simulink model "UKF"  (R2012b)
settings: Solver=ode4  StartTime=0.0  StopTime=SimulStop  FixedStep=T  RelTol=1e-3
values from neighbouring files (symbols this model uses):
  SimulStop = length(obv_traj1)*T    [parameter_IMM_UKF.m]
  T1 = 0.5    [parameter_IMM_UKF.m]
libraries: commnoisgen2 x1
settings Model: Creator=DonghanLee  LastModifiedBy=DonghanLee

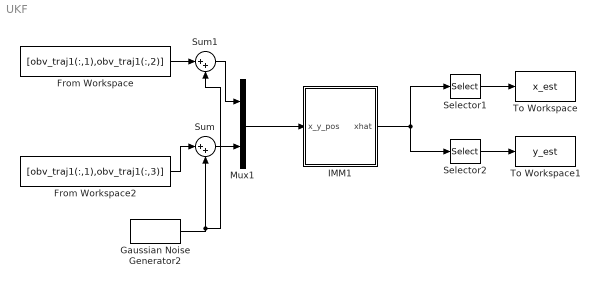
== system UKF ==
  From Workspace : FromWorkspace  VariableName=[obv_traj1(:,1),obv_traj1(:,2)]  SampleTime=0
  From Workspace2 : FromWorkspace  VariableName=[obv_traj1(:,1),obv_traj1(:,3)]  SampleTime=0
  Gaussian Noise Generator2 : commnoisgen2/Gaussian Noise Generator  m=0  d=noise  s=0  Ts=0.05  frameBased=off  sampPerFrame=1  orient=off  outDataType=double
  IMM1 : Subsystem
  Mux1 : Mux  Inputs=2
  Selector1 : Selector  InputPortWidth=5  IndexOptions=Index vector (dialog)  Indices=[1 2]  OutputSizes=1
  Selector2 : Selector  InputPortWidth=5  IndexOptions=Index vector (dialog)  Indices=[3 4]  OutputSizes=1
  Sum : Sum  Inputs=|++
  Sum1 : Sum  Inputs=|++
  To Workspace : ToWorkspace  VariableName=x_est  SampleTime=-1
  To Workspace1 : ToWorkspace  VariableName=y_est  SampleTime=-1
  wires:
  Gaussian Noise Generator2/1 -> Sum1/2, Sum/2
  From Workspace2/1 -> Sum/1
  Sum/1 -> Mux1/2
  From Workspace/1 -> Sum1/1
  Sum1/1 -> Mux1/1
  Mux1/1 -> IMM1/1(x_y_pos)
  IMM1/1(xhat) -> Selector2/1, Selector1/1
  Selector1/1 -> To Workspace/1
  Selector2/1 -> To Workspace1/1

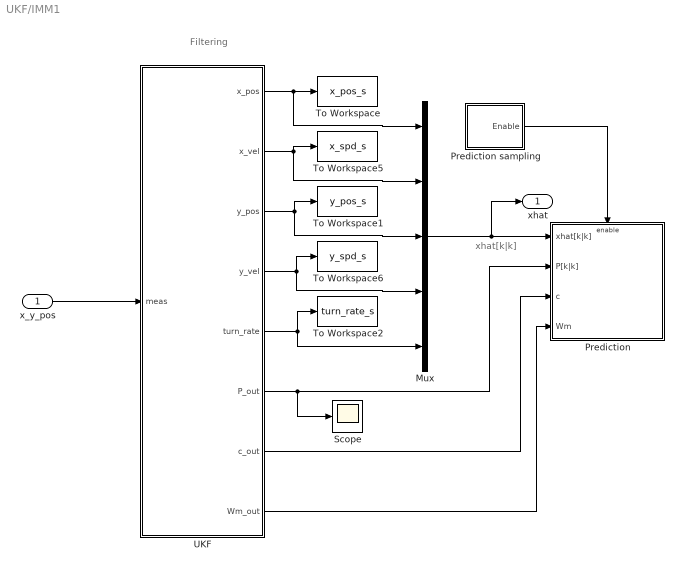
== system UKF/IMM1 ==
  note: xhat[k|k]
  note: Filtering
  x_y_pos : Inport
  Mux : Mux  Inputs=5
  Prediction : Subsystem
  Prediction sampling : Subsystem
  Scope : Scope
      settings: SaveName=ScopeData3
  To Workspace : ToWorkspace  VariableName=x_pos_s  SampleTime=-1
  To Workspace1 : ToWorkspace  VariableName=y_pos_s  SampleTime=-1
  To Workspace2 : ToWorkspace  VariableName=turn_rate_s  SampleTime=-1
  To Workspace5 : ToWorkspace  VariableName=x_spd_s  SampleTime=-1
  To Workspace6 : ToWorkspace  VariableName=y_spd_s  SampleTime=-1
  UKF : MATLAB Function  TreatAsAtomicUnit=on
  xhat : Outport
  wires:
  x_y_pos/1 -> UKF/1(meas)
  UKF/1(x_pos) -> Mux/1, To Workspace/1
  UKF/2(x_vel) -> To Workspace5/1, Mux/2
  UKF/3(y_pos) -> To Workspace1/1, Mux/3
  UKF/4(y_vel) -> To Workspace6/1, Mux/4
  UKF/5(turn_rate) -> To Workspace2/1, Mux/5
  Mux/1 -> xhat/1, Prediction/1(xhat[k|k])
  Prediction sampling/1(Enable) -> Prediction/Enable
  UKF/6(P_out) -> Prediction/2(P[k|k]), Scope/1
  UKF/7(c_out) -> Prediction/3(c)
  UKF/8(Wm_out) -> Prediction/4(Wm)

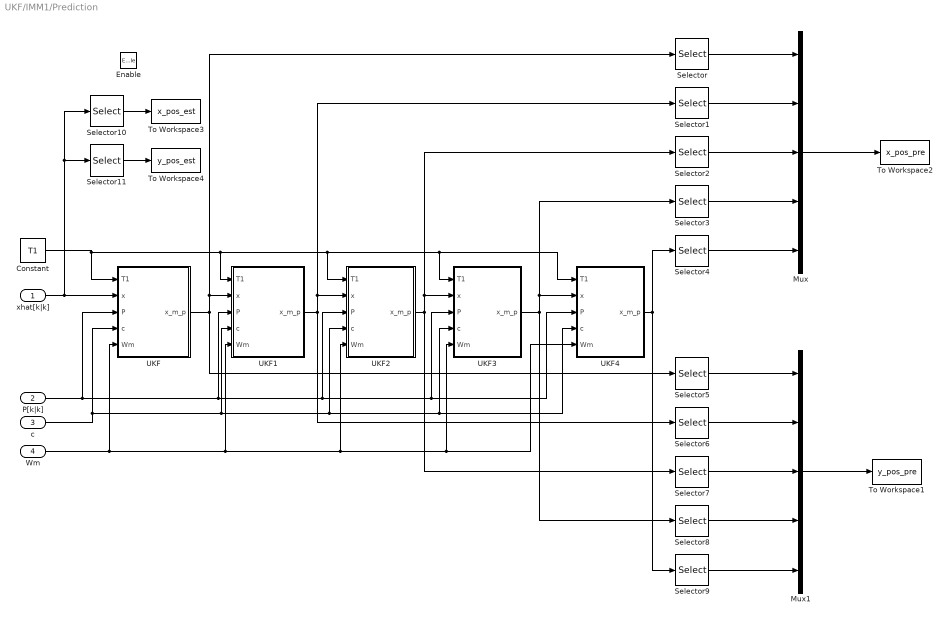
== system UKF/IMM1/Prediction ==
  xhat[k|k] : Inport
  P[k|k] : Inport  Port=2
  c : Inport  Port=3
  Wm : Inport  Port=4
  Enable : EnablePort
  Constant : Constant  Value=T1
  Mux : Mux  Inputs=5
  Mux1 : Mux  Inputs=5
  Selector{,1..4,10} (6 alike) : Selector  InputPortWidth=5  IndexOptions=Index vector (dialog)  Indices=[1]  OutputSizes=1
  Selector{5..9,11} (6 alike) : Selector  InputPortWidth=5  IndexOptions=Index vector (dialog)  Indices=[3]  OutputSizes=1
  To Workspace1 : ToWorkspace  VariableName=y_pos_pre  SampleTime=-1
  To Workspace2 : ToWorkspace  VariableName=x_pos_pre  SampleTime=-1
  To Workspace3 : ToWorkspace  VariableName=x_pos_est  SampleTime=-1
  To Workspace4 : ToWorkspace  VariableName=y_pos_est  SampleTime=-1
  UKF : MATLAB Function  TreatAsAtomicUnit=on
  UKF1 : MATLAB Function  TreatAsAtomicUnit=on
  UKF2 : MATLAB Function  TreatAsAtomicUnit=on
  UKF3 : MATLAB Function  TreatAsAtomicUnit=on
  UKF4 : MATLAB Function  TreatAsAtomicUnit=on
  wires:
  Mux/1 -> To Workspace2/1
  Mux1/1 -> To Workspace1/1
  Selector/1 -> Mux/1
  xhat[k|k]/1 -> UKF/2(x), Selector10/1, Selector11/1
  UKF/1(x_m_p) -> Selector5/1, UKF1/2(x), Selector/1
  UKF1/1(x_m_p) -> Selector6/1, UKF2/2(x), Selector1/1
  UKF2/1(x_m_p) -> Selector7/1, UKF3/2(x), Selector2/1
  UKF3/1(x_m_p) -> Selector8/1, UKF4/2(x), Selector3/1
  UKF4/1(x_m_p) -> Selector9/1, Selector4/1
  Selector2/1 -> Mux/3
  Selector4/1 -> Mux/5
  Selector1/1 -> Mux/2
  Selector3/1 -> Mux/4
  Selector6/1 -> Mux1/2
  Selector8/1 -> Mux1/4
  Selector5/1 -> Mux1/1
  Selector7/1 -> Mux1/3
  Selector9/1 -> Mux1/5
  Selector10/1 -> To Workspace3/1
  Selector11/1 -> To Workspace4/1
  P[k|k]/1 -> UKF1/3(P), UKF2/3(P), UKF4/3(P), UKF3/3(P), UKF/3(P)
  c/1 -> UKF1/4(c), UKF2/4(c), UKF4/4(c), UKF3/4(c), UKF/4(c)
  Wm/1 -> UKF1/5(Wm), UKF2/5(Wm), UKF4/5(Wm), UKF3/5(Wm), UKF/5(Wm)
  Constant/1 -> UKF1/1(T1), UKF2/1(T1), UKF4/1(T1), UKF3/1(T1), UKF/1(T1)

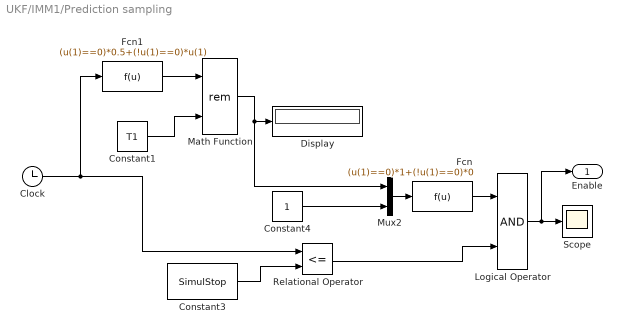
== system UKF/IMM1/Prediction sampling ==
  Clock : Clock
  Constant1 : Constant  Value=T1
  Constant3 : Constant  Value=SimulStop
  Constant4 : Constant
  Display : Display
  Fcn : Fcn  Expr=(u(1)==0)*1+(!u(1)==0)*0
  Fcn1 : Fcn  Expr=(u(1)==0)*0.5+(!u(1)==0)*u(1)
  Logical Operator : Logic  AllPortsSameDT=off  OutDataTypeStr=boolean
  Math Function : Math  Operator=rem  SaturateOnIntegerOverflow=on
  Mux2 : Mux  Inputs=2
  Relational Operator : RelationalOperator  Operator=<=  OutDataTypeStr=boolean
  Scope : Scope
      settings: SaveName=ScopeData2
  Enable : Outport
  wires:
  Clock/1 -> Fcn1/1, Relational Operator/1
  Constant1/1 -> Math Function/2
  Math Function/1 -> Mux2/1, Display/1
  Logical Operator/1 -> Enable/1, Scope/1
  Fcn/1 -> Logical Operator/1
  Relational Operator/1 -> Logical Operator/2
  Constant3/1 -> Relational Operator/2
  Constant4/1 -> Mux2/2
  Mux2/1 -> Fcn/1
  Fcn1/1 -> Math Function/1

== matlab function UKF/IMM1/UKF ==
  data: meas input; x_pos output; x_vel output; y_pos output; y_vel output; turn_rate output; P_out output; c_out output; Wm_out output
function [x_pos,x_vel,y_pos,y_vel,turn_rate,P_out,c_out,Wm_out] = UKF(meas)
% Define parametersInitialization
T=0.05; % Sampling time [s]
L=5; % Dimension of state vector
% Scaling Factors & Weights
alpha=0.001;                                 %default, tunable
kappa=0;                                       %default, tunable
beta=2;                                     %default, tunable

lambda=alpha^2*(L+kappa)-L;                    %scaling factor
c=L+lambda;                                 %scaling factor
% Wm=[lambda/c 0.5/c*ones(1,2*L)];           %weights for means
% Wc=Wm;
% Wc(1)=Wc(1)+(1-alpha^2+beta);               %weights for covariance

Wm = ones(2*L + 1,1)*1/(2*(L+lambda));
Wc = Wm;
Wm(1) = lambda/(lambda+L);
Wc(1) = lambda/(lambda+L) + 1 - alpha^2 + beta;
c=sqrt(c);

H = [1 0 0 0 0;
     0 0 1 0 0];

% Initialize
persistent P x W1 V1
if isempty(P)
% meas_noise1 = 0.5; 
% a_process_noise = 5*10^(-3); 
% w_process_noise = 5*10^(-4);  

meas_noise1 = 1.5;     % New freezed value
a_process_noise = 1.5*10^(-2); 
w_process_noise = 1.5*10^(-3); 

Sv1 = meas_noise1^2;
Sw1 = a_process_noise^2;
Sw2 = w_process_noise^2;
Sw = [Sw1 0 0;0 Sw1 0;0 0 Sw2];
%Bw = [0.5*T^2 0 0;T 0 0;0 0.5*T^2 0;0 T 0;0 0 T];

Bw = [T 0 0;1 0 0;0 T 0;0 1 0;0 0 1];

Dw = eye(2);
W1 = Bw*Sw*Bw';
V1 = Dw*Sv1*Dw';

P = eye(5,5);
x = zeros(L, 2*L+1);
x(:,1) = [meas(1,1);10^(-5);meas(2,1);0;10^(-5)];
%x(:,1) = [meas(1,1);10;meas(2,1);0;10^(-5)];

%y = zeros(L, 2*L+1);
end
% Generate sigma points
sP = chol(P,'lower');
chi_p = [x(:,1) x(:,1)*ones(1,L)+c*sP x(:,1)*ones(1,L)-c*sP];

% Prediction 
    chi_m = zeros(L,2*L+1);
    for i=1:2*L+1        
        chi_m(1,i) = chi_p(1,i)+ chi_p(2,i)*sin(chi_p(5,i)*T)/chi_p(5,i)-chi_p(4,i)*(1-cos(chi_p(5,i)*T))/chi_p(5,i);
        chi_m(2,i) = cos(chi_p(5,i)*T)*chi_p(2,i)-sin(chi_p(5,i)*T)*chi_p(4,i);
        chi_m(3,i) = chi_p(2,i)*(1-cos(chi_p(5,i)*T))/chi_p(5,i)+chi_p(3,i)+chi_p(4,i)*sin(chi_p(5,i)*T)/chi_p(5,i);
        chi_m(4,i) = chi_p(2,i)*sin(chi_p(5,i)*T)+chi_p(4,i)*cos(chi_p(5,i)*T);
        chi_m(5,i) = chi_p(5,i);
    end        
    x_m = chi_m*Wm;    
    P_m = W1;
    for i=1:2*L+1
        P_m = P_m+Wc(i)*(chi_m(:,i)-x_m)*(chi_m(:,i)-x_m)';
    end
    psi_m = H*chi_m;
    y_m = psi_m*Wm;
    
% Update
    Pyy = V1;
    Pxy = zeros(L,2);
    for i=1:2*L+1
        Pyy = Pyy+Wc(i)*(psi_m(:,i)-y_m)*(psi_m(:,i)-y_m)';
        Pxy = Pxy+Wc(i)*(chi_m(:,i)-x_m)*(psi_m(:,i)-y_m)';
    end
    
    K = Pxy*inv(Pyy);
    x(:,1) = x_m + K*(meas - y_m);
    P = P_m-K*Pyy*K';

% Post the results
x_pos = x(1,1);
x_vel = x(2,1);
y_pos = x(3,1);
y_vel = x(4,1);
turn_rate = x(5,1);
P_out=P;   
c_out = c;
Wm_out = Wm;

== matlab function UKF/IMM1/Prediction/UKF ==
  data: T1 input; x input; x_m_p output; P input; c input; Wm input
function x_m_p  = UKF_pred(T1,x,P,c,Wm)
L=5;
sP = chol(P,'lower');
chi_p = [x(:,1) x(:,1)*ones(1,L)+c*sP x(:,1)*ones(1,L)-c*sP];

% Prediction 
    chi_m_p = zeros(L,2*L+1);
    for i=1:2*L+1        
        chi_m_p(1,i) = chi_p(1,i)+ chi_p(2,i)*sin(chi_p(5,i)*T1)/chi_p(5,i)-chi_p(4,i)*(1-cos(chi_p(5,i)*T1))/chi_p(5,i);
        chi_m_p(2,i) = cos(chi_p(5,i)*T1)*chi_p(2,i)-sin(chi_p(5,i)*T1)*chi_p(4,i);
        chi_m_p(3,i) = chi_p(2,i)*(1-cos(chi_p(5,i)*T1))/chi_p(5,i)+chi_p(3,i)+chi_p(4,i)*sin(chi_p(5,i)*T1)/chi_p(5,i);
        chi_m_p(4,i) = chi_p(2,i)*sin(chi_p(5,i)*T1)+chi_p(4,i)*cos(chi_p(5,i)*T1);
        chi_m_p(5,i) = chi_p(5,i);
    end        
    x_m_p = chi_m_p*Wm;

== matlab function UKF/IMM1/Prediction/UKF1 ==
  data: T1 input; x input; x_m_p output; P input; c input; Wm input
function x_m_p  = UKF_pred(T1,x,P,c,Wm)
L=5;
sP = chol(P,'lower');
chi_p = [x(:,1) x(:,1)*ones(1,L)+c*sP x(:,1)*ones(1,L)-c*sP];

% Prediction 
    chi_m_p = zeros(L,2*L+1);
    for i=1:2*L+1        
        chi_m_p(1,i) = chi_p(1,i)+ chi_p(2,i)*sin(chi_p(5,i)*T1)/chi_p(5,i)-chi_p(4,i)*(1-cos(chi_p(5,i)*T1))/chi_p(5,i);
        chi_m_p(2,i) = cos(chi_p(5,i)*T1)*chi_p(2,i)-sin(chi_p(5,i)*T1)*chi_p(4,i);
        chi_m_p(3,i) = chi_p(2,i)*(1-cos(chi_p(5,i)*T1))/chi_p(5,i)+chi_p(3,i)+chi_p(4,i)*sin(chi_p(5,i)*T1)/chi_p(5,i);
        chi_m_p(4,i) = chi_p(2,i)*sin(chi_p(5,i)*T1)+chi_p(4,i)*cos(chi_p(5,i)*T1);
        chi_m_p(5,i) = chi_p(5,i);
    end        
    x_m_p = chi_m_p*Wm;

== matlab function UKF/IMM1/Prediction/UKF2 ==
  data: T1 input; x input; x_m_p output; P input; c input; Wm input
function x_m_p  = UKF_pred(T1,x,P,c,Wm)
L=5;
sP = chol(P,'lower');
chi_p = [x(:,1) x(:,1)*ones(1,L)+c*sP x(:,1)*ones(1,L)-c*sP];

% Prediction 
    chi_m_p = zeros(L,2*L+1);
    for i=1:2*L+1        
        chi_m_p(1,i) = chi_p(1,i)+ chi_p(2,i)*sin(chi_p(5,i)*T1)/chi_p(5,i)-chi_p(4,i)*(1-cos(chi_p(5,i)*T1))/chi_p(5,i);
        chi_m_p(2,i) = cos(chi_p(5,i)*T1)*chi_p(2,i)-sin(chi_p(5,i)*T1)*chi_p(4,i);
        chi_m_p(3,i) = chi_p(2,i)*(1-cos(chi_p(5,i)*T1))/chi_p(5,i)+chi_p(3,i)+chi_p(4,i)*sin(chi_p(5,i)*T1)/chi_p(5,i);
        chi_m_p(4,i) = chi_p(2,i)*sin(chi_p(5,i)*T1)+chi_p(4,i)*cos(chi_p(5,i)*T1);
        chi_m_p(5,i) = chi_p(5,i);
    end        
    x_m_p = chi_m_p*Wm;

== matlab function UKF/IMM1/Prediction/UKF3 ==
  data: T1 input; x input; x_m_p output; P input; c input; Wm input
function x_m_p  = UKF_pred(T1,x,P,c,Wm)
L=5;
sP = chol(P,'lower');
chi_p = [x(:,1) x(:,1)*ones(1,L)+c*sP x(:,1)*ones(1,L)-c*sP];

% Prediction 
    chi_m_p = zeros(L,2*L+1);
    for i=1:2*L+1        
        chi_m_p(1,i) = chi_p(1,i)+ chi_p(2,i)*sin(chi_p(5,i)*T1)/chi_p(5,i)-chi_p(4,i)*(1-cos(chi_p(5,i)*T1))/chi_p(5,i);
        chi_m_p(2,i) = cos(chi_p(5,i)*T1)*chi_p(2,i)-sin(chi_p(5,i)*T1)*chi_p(4,i);
        chi_m_p(3,i) = chi_p(2,i)*(1-cos(chi_p(5,i)*T1))/chi_p(5,i)+chi_p(3,i)+chi_p(4,i)*sin(chi_p(5,i)*T1)/chi_p(5,i);
        chi_m_p(4,i) = chi_p(2,i)*sin(chi_p(5,i)*T1)+chi_p(4,i)*cos(chi_p(5,i)*T1);
        chi_m_p(5,i) = chi_p(5,i);
    end        
    x_m_p = chi_m_p*Wm;

== matlab function UKF/IMM1/Prediction/UKF4 ==
  data: T1 input; x input; x_m_p output; P input; c input; Wm input
function x_m_p  = UKF_pred(T1,x,P,c,Wm)
L=5;
sP = chol(P,'lower');
chi_p = [x(:,1) x(:,1)*ones(1,L)+c*sP x(:,1)*ones(1,L)-c*sP];

% Prediction 
    chi_m_p = zeros(L,2*L+1);
    for i=1:2*L+1        
        chi_m_p(1,i) = chi_p(1,i)+ chi_p(2,i)*sin(chi_p(5,i)*T1)/chi_p(5,i)-chi_p(4,i)*(1-cos(chi_p(5,i)*T1))/chi_p(5,i);
        chi_m_p(2,i) = cos(chi_p(5,i)*T1)*chi_p(2,i)-sin(chi_p(5,i)*T1)*chi_p(4,i);
        chi_m_p(3,i) = chi_p(2,i)*(1-cos(chi_p(5,i)*T1))/chi_p(5,i)+chi_p(3,i)+chi_p(4,i)*sin(chi_p(5,i)*T1)/chi_p(5,i);
        chi_m_p(4,i) = chi_p(2,i)*sin(chi_p(5,i)*T1)+chi_p(4,i)*cos(chi_p(5,i)*T1);
        chi_m_p(5,i) = chi_p(5,i);
    end        
    x_m_p = chi_m_p*Wm;
